simulink model "I_O_FBL"  (R2022a)
settings: Solver=VariableStepAuto  StartTime=0.0  StopTime=25  MaxStep=1e-3  RelTol=1e-3
InitFcn:
  | clear
  | clc
  | %% dati
  | w0 = 5.278;
  | alfa1 = w0^2;
  | alfa3 = -1.402*w0^2;
  | alfa5 = 0.271*w0^2;
  | mu1 = 0.086;
  | mu3 = 0.1080;
  | %% disturbi e variazioni parametriche
  | Ad = 0;
  | fd = 2;
  | alfa1_hat = 0.8*w0^2;
libraries: slpidlib x1
settings Model: Creator=user  LastModifiedBy=user

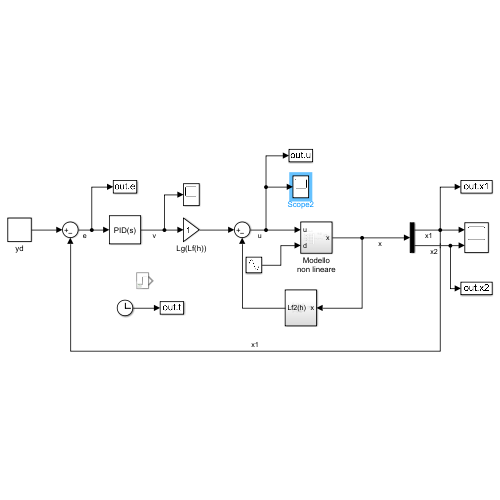
[thumbnail: Simulink's stored preview of the top-level diagram]
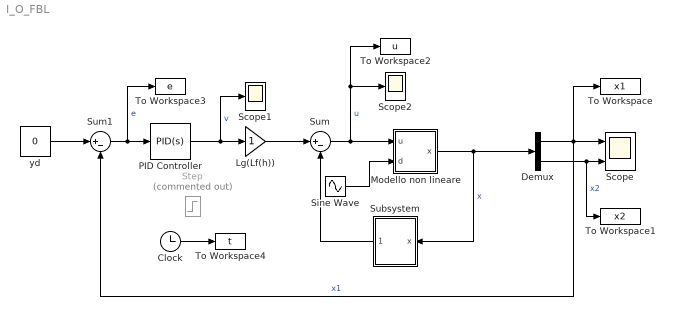
== system I_O_FBL ==
  Clock : Clock
  Demux : Demux  Outputs=2
  Lg(Lf(h)) : Gain
  Modello non lineare : Subsystem
  PID Controller : slpidlib/PID Controller  Controller=PID  Form=Parallel  TimeDomain=Continuous-time  UseExternalTs=off  SampleTime=-1  IntegratorMethod=Forward Euler  FilterMethod=Forward Euler  ControllerParametersSource=internal  P=3  I=3  UseKiTs=off  D=7  N=18  UseFilter=on  TunerSelectOption=Transfer Function Based (PID Tuner App)  InitialConditionSource=internal  InitialConditionForIntegrator=0  InitialConditionForFilter=0  DifferentiatorICPrevScaledInput=0  ExternalReset=none  TrackingMode=off  Kt=1  LimitOutput=off  SatLimitsSource=internal  UpperSaturationLimit=inf  LowerSaturationLimit=-inf  LinearizeAsGain=on  AntiWindupMode=none  Kb=1  POutMin=[]  POutMax=[]  IOutMin=[]  IOutMax=[]  DOutMin=[]  DOutMax=[]  NOutMin=[]  NOutMax=[]  SumOutMin=[]  SumOutMax=[]  SaturationOutMin=[]  SaturationOutMax=[]  PParamMin=[]  PParamMax=[]  IParamMin=[]  IParamMax=[]  DParamMin=[]  DParamMax=[]  NParamMin=[]  NParamMax=[]  KbParamMin=[]  KbParamMax=[]  KtParamMin=[]  KtParamMax=[]  KbOutMin=[]  KbOutMax=[]  KtOutMin=[]  KtOutMax=[]  IntegratorOutMin=[]  IntegratorOutMax=[]  FilterOutMin=[]  FilterOutMax=[]  SumI1OutMin=[]  SumI1OutMax=[]  SumI2OutMin=[]  SumI2OutMax=[]  SumI3OutMin=[]  SumI3OutMax=[]  SumI4OutMin=[]  SumI4OutMax=[]  SumDOutMin=[]  SumDOutMax=[]  DifferentiatorOutMin=[]  DifferentiatorOutMax=[]  FilterDiffOutCoefMin=[]  FilterDiffOutCoefMax=[]  ReciprocalOutMin=[]  ReciprocalOutMax=[]  SumDenOutMin=[]  SumDenOutMax=[]  SumNumOutMin=[]  SumNumOutMax=[]  DivideOutMin=[]  DivideOutMax=[]  UdiffTsProdOutMin=[]  UdiffTsProdOutMax=[]  NTsProdOutMin=[]  NTsProdOutMax=[]  UintegralTsProdOutMin=[]  UintegralTsProdOutMax=[]  UngainTsProdOutMin=[]  UngainTsProdOutMax=[]  IntegratorContinuousStateAttributes=''  IntegratorStateMustResolveToSignalObject=off  IntegratorRTWStateStorageClass=Auto  FilterContinuousStateAttributes=''  FilterStateMustResolveToSignalObject=off  FilterRTWStateStorageClass=Auto  ParallelPVariant=InternalParameters  IdealPVariant=Disabled  IVariant=InternalParameters  DVariant=InternalParameters  IntegratorVariant=Continuous  SatVariant=Disabled  AWVariant=Passthrough  PCopyVariant=Disabled  TRVariant=Disabled  FdbkBlocksVariant=Forward  IdealPFdbkVariant=Disabled  SatFdbkVariant=Disabled  DerivativeFilterVariant=ContFilter  NVariant=InternalParameters  NCopyVariant=Disabled  FilterICVariant=InternalICsFilter  IntegratorICVariant=InternalICs  ExternalResetVariant=Disabled  TRSumVariant=Passthrough  SumFdbkVariant=Disabled  SumVariant=Sum_PID  TsampFilterVariant=InternalTs  TsampNgainVariant=Passthrough  TsampIntegralVariant=Passthrough  ExternalSaturationOutDataTypeStr=Inherit: Same as second input  aMode=0
  Scope : Scope  NumInputPorts=2
  Scope1 : Scope
  Scope2 : Scope
  Sine Wave : Sin  Amplitude=Ad  Frequency=fd  SampleTime=0
  Step : Step  Commented=on  Time=20  After=2  SampleTime=0
  Subsystem : Subsystem
  Sum : Sum  Inputs=|+-
  Sum1 : Sum  Inputs=|+-
  To Workspace : ToWorkspace  VariableName=x1  SampleTime=-1
      settings: Save2DSignal=2-D array (concatenate along first dimension)
  To Workspace1 : ToWorkspace  VariableName=x2  SampleTime=-1
      settings: Save2DSignal=2-D array (concatenate along first dimension)
  To Workspace2 : ToWorkspace  VariableName=u  SampleTime=-1
      settings: Save2DSignal=2-D array (concatenate along first dimension)
  To Workspace3 : ToWorkspace  VariableName=e  SampleTime=-1
      settings: Save2DSignal=2-D array (concatenate along first dimension)
  To Workspace4 : ToWorkspace  VariableName=t  SampleTime=-1
      settings: Save2DSignal=2-D array (concatenate along first dimension)
  yd : Constant  Value=0
  wires:
  Sum/1 -> To Workspace2/1, Scope2/1, Modello non lineare/1(u)  "u"
  Lg(Lf(h))/1 -> Sum/1
  Modello non lineare/1(x) -> Subsystem/1(x), Demux/1  "x"
  Subsystem/1(Lf2(h)) -> Sum/2
  PID Controller/1 -> Scope1/1, Lg(Lf(h))/1  "v"
  Demux/1 -> To Workspace/1, Scope/1, Sum1/2  "x1"
  Demux/2 -> Scope/2, To Workspace1/1  "x2"
  Sum1/1 -> To Workspace3/1, PID Controller/1  "e"
  yd/1 -> Sum1/1
  Clock/1 -> To Workspace4/1
  Sine Wave/1 -> Modello non lineare/2(d)

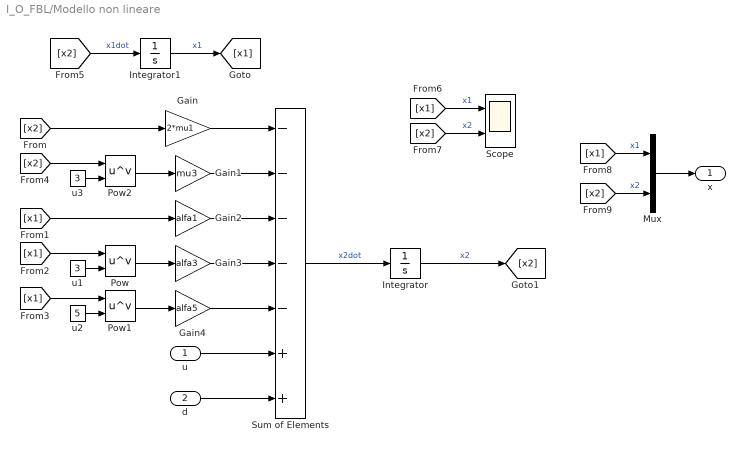
== system I_O_FBL/Modello non lineare ==
  u : Inport
  d : Inport  Port=2
  Gain : Gain  Gain=2*mu1
  Gain1 : Gain  Gain=mu3
  Gain2 : Gain  Gain=alfa1
  Gain3 : Gain  Gain=alfa3
  Gain4 : Gain  Gain=alfa5
  Integrator : Integrator  InitialCondition=-0.18
  Integrator1 : Integrator  InitialCondition=-1.2
  Mux : Mux  Inputs=2
  Pow : Math  Operator=pow  RndMeth=Zero
  Pow1 : Math  Operator=pow  RndMeth=Zero
  Pow2 : Math  Operator=pow  RndMeth=Zero
  Scope : Scope  NumInputPorts=2
  Sum of Elements : Sum  Inputs=-----++
  u1 : Constant  Value=3
  u2 : Constant  Value=5
  u3 : Constant  Value=3
  x : Outport
  wires:
  Gain/1 -> Sum of Elements/1
  [x2] -> Integrator1/1  "x1dot"
  [x1] -> Pow/1
  u2/1 -> Pow1/2
  Integrator/1 -> [x2]  "x2"
  Sum of Elements/1 -> Integrator/1  "x2dot"
  Gain4/1 -> Sum of Elements/5
  Integrator1/1 -> [x1]  "x1"
  Pow2/1 -> Gain1/1
  [x1] -> Gain2/1
  Gain3/1 -> Sum of Elements/4
  u3/1 -> Pow2/2
  Gain1/1 -> Sum of Elements/2
  Pow/1 -> Gain3/1
  [x1] -> Pow1/1
  u1/1 -> Pow/2
  Pow1/1 -> Gain4/1
  Gain2/1 -> Sum of Elements/3
  [x2] -> Pow2/1
  [x2] -> Scope/2  "x2"
  [x2] -> Gain/1
  [x1] -> Scope/1  "x1"
  u/1 -> Sum of Elements/6
  [x1] -> Mux/1  "x1"
  [x2] -> Mux/2  "x2"
  Mux/1 -> x/1
  d/1 -> Sum of Elements/7

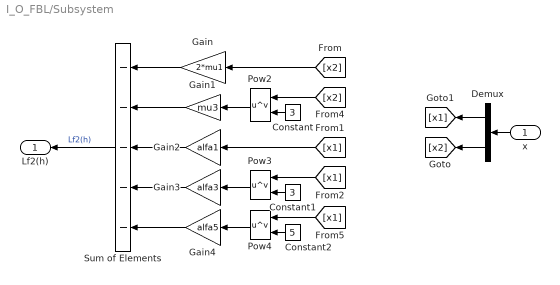
== system I_O_FBL/Subsystem ==
  x : Inport
  Constant : Constant  Value=3
  Constant1 : Constant  Value=3
  Constant2 : Constant  Value=5
  Demux : Demux  Outputs=2
  Gain : Gain  Gain=2*mu1
  Gain1 : Gain  Gain=mu3
  Gain2 : Gain  Gain=alfa1
  Gain3 : Gain  Gain=alfa3
  Gain4 : Gain  Gain=alfa5
  Pow2 : Math  Operator=pow  RndMeth=Zero
  Pow3 : Math  Operator=pow  RndMeth=Zero
  Pow4 : Math  Operator=pow  RndMeth=Zero
  Sum of Elements : Sum  Inputs=-----
  Lf2(h) : Outport
  wires:
  Gain/1 -> Sum of Elements/1
  Constant1/1 -> Pow3/2
  [x2] -> Pow2/1
  Pow3/1 -> Gain3/1
  Gain3/1 -> Sum of Elements/4
  Pow2/1 -> Gain1/1
  Gain1/1 -> Sum of Elements/2
  Gain2/1 -> Sum of Elements/3
  [x2] -> Gain/1
  [x1] -> Pow3/1
  Gain4/1 -> Sum of Elements/5
  [x1] -> Pow4/1
  Constant/1 -> Pow2/2
  Constant2/1 -> Pow4/2
  Sum of Elements/1 -> Lf2(h)/1  "Lf2(h)"
  Pow4/1 -> Gain4/1
  [x1] -> Gain2/1
  Demux/2 -> [x2]
  Demux/1 -> [x1]
  x/1 -> Demux/1
